simulink model "modelo_planta"  (R2023b)
settings: Solver=VariableStepAuto  StartTime=0.0  StopTime=inf  MaxStep=1e-3  RelTol=1e-3
undefined symbols (not defined in the file): ah_max, at_max, bcx, bcy, bhb, bhd, bhEb, bhm, bhwu, bt, btb, btd, btm, btw, DiscIntNeverNeededParam, g, h_vec_inicial, Hc, ih, it, J_hd_hEb, J_hm_hb, Jtd, Jtm_tb, Kcy, khwu, Ki_h, Ki_t, Kp_h, Kp_t, Kpos_h, Kpos_t, Ktw, lambda, Lh0, lh_0, magnitude, Mc_max, Mc_min, Ms, Mt, P_nom, rhd, rtd, tau_hm, tau_tm, Thb_Max, ThEb_Max, Thm_0, Thm_Max, titahm_0, titatm_0, Ts0, Ts1, Ts2, Ttb_Max, Ttm_0, Ttm_Max, vh_max_unloaded, vh_nom ... (+20)
libraries: simulink x14, vrlib x1, simulink_extras x1, dspnetwork x1
(part 1 of 2)
settings Model: PacingRate=0.500000  Creator=Nahuel  LastModifiedBy=rodri
settings SolverCC: ZeroCrossControl=DisableAll
settings DebuggingCC: UnderSpecifiedDimensionMsg=warning

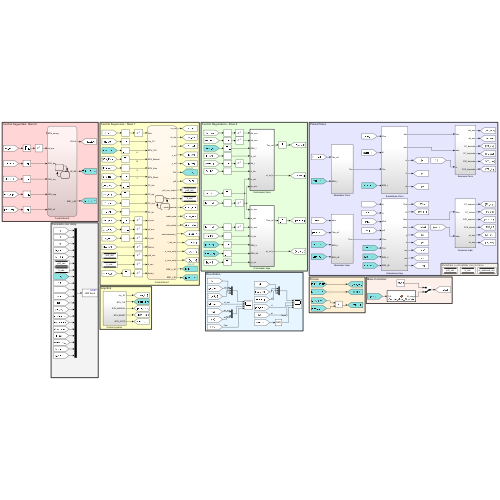
[thumbnail: Simulink's stored preview of the top-level diagram]
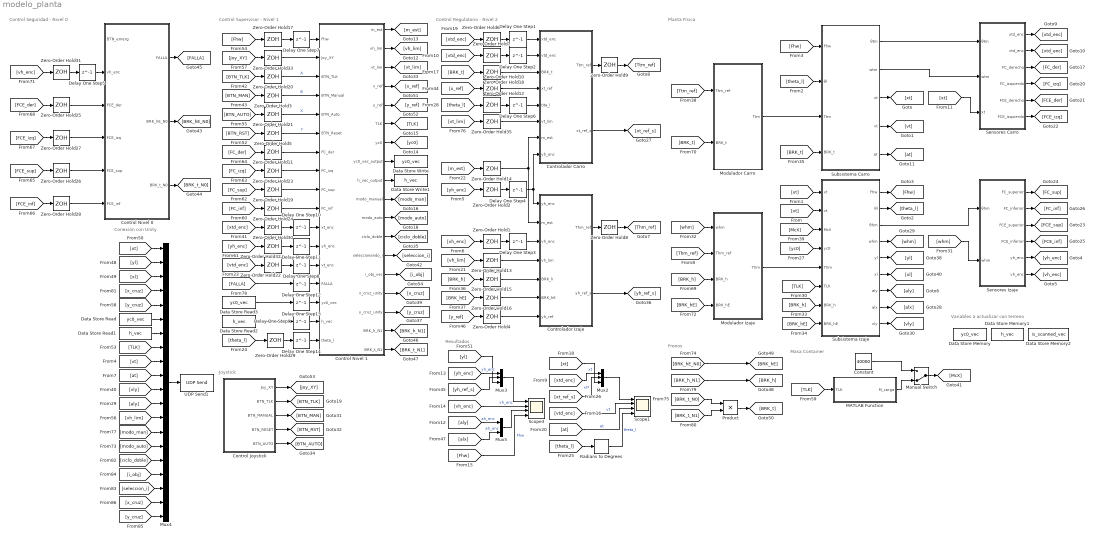
== system modelo_planta ==
  note: Joystick
  note: Frenos
  note: Control Seguridad - Nivel 0
  note: Control Regulatorio - Nivel 2
  note: Control Supervisor - Nivel 1
  note: Conexión con Unity
  note: Planta Física
  note: Resultados
  note: Variables a actualizar con terreno
  note: Masa Container
  Constant : Constant  Value=40000
  "Control Joystick " : Subsystem
  Control Nivel 0 : Stateflow chart  TreatAsAtomicUnit=on
      settings: PortSchema="{\"entries\":[{\"content\":{\"sides\":[{\"content\":{\"connectorIds\":[\"In1\",\"In4\",\"In2\",\"In5\",\"In3\",\"In6\"]},\"type\":\"ConnectorPlacement.EquallySpacedRectSide\",\"uuid\":\"72248b79-25cb-4c81-9f00-8922a9a1cf34\"},{\"content\":{\"connectorIds\":[\"Out1\",\"Out2\",\"Out3\"],\"side\":\"RIGHT\"},\"type\":\"ConnectorPlacement.EquallySpacedRectSide\",\"uuid\":\"f4bfcd12-c204-46a9-9a4b-20ccb9bfcfbb\"},{\"content\":{\"side\":\"TOP\"},\"type\":\"ConnectorPlacement.EquallySpacedRectSide\",\"uuid\":\"f84291a0-0f0e-4f0d-b220-c2febce5b448\"}]},\"type\":\"ConnectorPlacement.EquallySpacedConnector\",\"uuid\":\"3b165743-ae9e-4544-8961-e71410288a4b\"}],\"packageUris\":[\"http://schema.mathworks.com/mf0/Connector/R2020b\"],\"version\":\"1.0\"}"
  Control Nivel 1 : Stateflow chart  TreatAsAtomicUnit=on
      settings: PortSchema="{\"entries\":[{\"content\":{\"sides\":[{\"content\":{\"connectorIds\":[\"In2\",\"In4\",\"In3\",\"In5\",\"In6\",\"In7\",\"In8\",\"In10\",\"In9\",\"In11\",\"In12\",\"In13\",\"In1\",\"In14\",\"In15\",\"In16\",\"In17\"]},\"type\":\"ConnectorPlacement.EquallySpacedRectSide\",\"uuid\":\"72765c9f-68bf-44f3-92f3-3edecb9ca866\"},{\"content\":{\"connectorIds\":[\"Out1\",\"Out2\",\"Out7\",\"Out3\",\"Out4\",\"Out8\",\"Out9\",\"Out10\",\"Out11\",\"Out12\",\"Out13\",\"Out14\",\"Out15\",\"Out16\",\"Out17\",\"Out18\",\"Out5\",\"Out6\"],\"side\":\"RIGHT\"},\"type\":\"ConnectorPlacement.EquallySpacedRectSide\",\"uuid\":\"a6939ff5-eef8-44e2-80ea-5356e254e9e8\"},{\"content\":{\"side\":\"TOP\"},\"type\":\"ConnectorPlacement.EquallySpacedRectSide\",\"uuid\":\"0bd5f797-ecd4-419a-b4ec-9e10260d270a\"},{\"content\":{\"side\":\"BOTTOM\"},\"type\":\"ConnectorPlacement.EquallySpacedRectSide\",\"uuid\":\"7945275f-dab8-4c32-b5c3-f64b82fddda0\"}]},\"type\":\"ConnectorPlacement.EquallySpacedConnector\",\"uuid\":\"3d3cbadb-c70b-461a-afd4-e8d4b160ddcd\"}],\"packageUris\":[\"http://schema.mathworks.com/mf0/Connector/R2020b\"],\"version\":\"1.0\"}"
  Controlador Carro : Subsystem  TreatAsAtomicUnit=on  SystemSampleTime=Ts2
  Controlador Izaje : Subsystem  TreatAsAtomicUnit=on  SystemSampleTime=Ts2
  Data Store Memory : DataStoreMemory  DataStoreName=yc0_vec  WriteAfterWriteMsg=warning  InitialValue=yc0_vec_inicial  ShowAdditionalParam=off  OutDataTypeStr=double
  Data Store Memory1 : DataStoreMemory  DataStoreName=h_vec  WriteAfterWriteMsg=warning  InitialValue=h_vec_inicial  ShowAdditionalParam=off  OutDataTypeStr=double  Dimensions=[1,33]
  Data Store Memory2 : DataStoreMemory  DataStoreName=is_scanned_vec  WriteAfterWriteMsg=warning  InitialValue=is_scanned_vec  ShowAdditionalParam=off
  Data Store Read : DataStoreRead  DataStoreName=yc0_vec  IndexOptions=Index vector (dialog)  Indices=1  OutputSizes=1
  Data Store Read1 : DataStoreRead  DataStoreName=h_vec  IndexOptions=Index vector (dialog)  Indices=1  OutputSizes=1
  Data Store Read2 : DataStoreRead  DataStoreName=h_vec  IndexOptions=Index vector (dialog)  Indices=1  OutputSizes=1
  Data Store Read3 : DataStoreRead  DataStoreName=yc0_vec  IndexOptions=Index vector (dialog)  Indices=1  OutputSizes=1
  Data Store Write : DataStoreWrite  DataStoreName=yc0_vec  IndexOptions=Index vector (dialog)  Indices=1  OutputSizes=1
  Data Store Write1 : DataStoreWrite  DataStoreName=h_vec  IndexOptions=Index vector (dialog)  Indices=1  OutputSizes=1
  Delay One Step1 : Delay  DelayLength=1  InitialCondition=xt_0
  Delay One Step10 : Delay  DelayLength=1  InitialCondition=xt_0
  Delay One Step11 : Delay  DelayLength=1  InitialCondition=yh_0
  Delay One Step12 : Delay  DelayLength=1
  Delay One Step13 : Delay  DelayLength=1  InitialCondition=yc0_vec_inicial
  Delay One Step14 : Delay  DelayLength=1  InitialCondition=0
  Delay One Step2 : Delay  DelayLength=1  InitialCondition=vt_0
  Delay One Step3 : Delay  DelayLength=1  InitialCondition=whm_0
  Delay One Step4 : Delay  DelayLength=1  InitialCondition=yh_0
  Delay One Step5 : Delay  DelayLength=1  InitialCondition=yh_0
  Delay One Step6 : Delay  DelayLength=1  InitialCondition=0
  Delay One Step7 : Delay  DelayLength=1
  Delay One Step8 : Delay  DelayLength=1  InitialCondition=0
  Delay One Step9 : Delay  DelayLength=1  InitialCondition=h_vec_inicial
  MATLAB Function : MATLAB Function  TreatAsAtomicUnit=on
  Manual Switch : ManualSwitch  CurrentSetting=0
  Modulador Carro : Subsystem
  Modulador Izaje : Subsystem
  Mux2 : Mux  Inputs=3
  Mux3 : Mux  Inputs=3
  Mux4 : Mux  Inputs=20
  Mux5 : Mux  Inputs=2
  Product : Product
  Radians to Degrees : simulink_extras/Transformations/Radians to Degrees
  Scope1 : Scope  NumInputPorts=4
  Scope3 : Scope  NumInputPorts=4
  Sensores Carro : Subsystem
  Sensores Izaje : Subsystem
  Subsistema Carro : Subsystem
  Subsistema Izaje : Subsystem
  UDP Send1 : dspnetwork/UDP Send  remoteURL='127.0.0.1'  remotePort=1234  localURL='0.0.0.0'  localPortSource=Automatically determine  localPort=-1  sendBufferSize=8192  sampletime=-1  blockPlatform=HOST  separateLengthPort=0
  Zero-Order Hold{1..2,4,6..10,12..16,18,35} (15 alike) : ZeroOrderHold  SampleTime=Ts2
  Zero-Order Hold{3,5,11,17,19..24,29..30,32..33} (14 alike) : ZeroOrderHold  SampleTime=Ts1
  Zero-Order Hold{25..28,31} (5 alike) : ZeroOrderHold  SampleTime=Ts0
  wires:
  [Thm_ref] -> Modulador Izaje/2(Thm_ref)
  [vh_enc] -> Scope3/2  "vh_enc"
  Sensores Izaje/2(FC_inferior) -> [FC_inf]
  [x_ref] -> Zero-Order Hold10/1
  Zero-Order Hold4/1 -> Controlador Izaje/7(yh_ref)
  Delay One Step4/1 -> Controlador Izaje/1(yh_enc), Controlador Carro/8(yh_enc)
  Sensores Izaje/5(yh_enc) -> [yh_enc]
  [BRK_hE] -> Subsistema Izaje/8(BRK_hE)
  Subsistema Izaje/1(Fhw) -> [Fhw]
  [vh_enc] -> Zero-Order Hold1/1
  Controlador Izaje/1(Thm_ref) -> Zero-Order Hold8/1
  Sensores Carro/1(xtd_enc) -> [xtd_enc]
  [xt] -> Sensores Carro/3(xt)
  [BRK_h] -> Subsistema Izaje/7(BRK_h)
  Sensores Carro/4(FC_izquierdo) -> [FC_izq]
  Subsistema Izaje/4(whm) -> [whm]
  [m_est] -> Zero-Order Hold14/1
  Controlador Carro/2(xt_ref_s) -> [xt_ref_s]
  Zero-Order Hold1/1 -> Delay One Step3/1
  Zero-Order Hold2/1 -> Delay One Step4/1
  Zero-Order Hold6/1 -> Delay One Step1/1
  Subsistema Carro/2(wtm) -> Sensores Carro/2(wtm)
  Subsistema Carro/5(at) -> [at]
  [theta_l] -> Subsistema Carro/2(θl)
  [vt] -> Subsistema Izaje/2(vt)
  [xt] -> Subsistema Izaje/1(xt)
  Delay One Step1/1 -> Controlador Carro/1(xtd_enc)
  [aly] -> Mux5/1  "ah_enc"
  [vtd_enc] -> Zero-Order Hold7/1
  Sensores Carro/2(vtd_enc) -> [vtd_enc]
  Zero-Order Hold8/1 -> [Thm_ref]
  Delay One Step3/1 -> Controlador Izaje/3(vh_enc)
  [vh_lim] -> Zero-Order Hold13/1
  Delay One Step2/1 -> Controlador Carro/2(vtd_enc)
  Zero-Order Hold10/1 -> Controlador Carro/4(xt_ref)
  Subsistema Carro/3(xt) -> [xt]
  [Fhw] -> Subsistema Carro/1(Fhw)
  Sensores Carro/6(FCE_izquierdo) -> [FCE_izq]
  [yh_enc] -> Zero-Order Hold2/1
  Sensores Izaje/6(vh_enc) -> [vh_enc]
  [xtd_enc] -> Zero-Order Hold6/1
  Zero-Order Hold9/1 -> [Ttm_ref]
  Controlador Carro/1(Ttm_ref) -> Zero-Order Hold9/1
  [TLK] -> Subsistema Izaje/6(TLK)
  Subsistema Izaje/3(θhm) -> Sensores Izaje/1(θhm)
  Subsistema Carro/1(θtm) -> Sensores Carro/1(θtm)
  Sensores Izaje/4(FCE_inferior) -> [FCE_inf]
  Sensores Izaje/3(FCE_superior) -> [FCE_sup]
  Sensores Izaje/1(FC_superior) -> [FC_sup]
  Sensores Carro/5(FCE_derecho) -> [FCE_der]
  Zero-Order Hold7/1 -> Delay One Step2/1
  Subsistema Izaje/2(θl) -> [theta_l]
  [McX] -> Subsistema Izaje/3(McX)
  Subsistema Carro/4(vt) -> [vt]
  Sensores Carro/3(FC_derecho) -> [FC_der]
  [whm] -> Sensores Izaje/2(whm)
  [BRK_t] -> Subsistema Carro/4(BRK_t)
  [BRK_h] -> Zero-Order Hold15/1
  [BRK_hE] -> Zero-Order Hold16/1
  [Ttm_ref] -> Modulador Carro/1(Ttm_ref)
  [BRK_t] -> Zero-Order Hold18/1
  [yh_enc] -> Mux3/1  "yh_enc"
  [whm] -> Modulador Izaje/1(whm)
  Delay One Step6/1 -> Controlador Carro/5(tita_l)
  [theta_l] -> Zero-Order Hold12/1
  Zero-Order Hold12/1 -> Delay One Step6/1
  Modulador Izaje/1(Thm) -> Subsistema Izaje/5(Thm)
  Modulador Carro/1(Ttm) -> Subsistema Carro/3(Ttm)
  [y_ref] -> Zero-Order Hold4/1
  Mux3/1 -> Scope3/1
  Controlador Izaje/2(yh_ref_s) -> [yh_ref_s]
  [yh_ref_s] -> Mux3/2
  Subsistema Izaje/5(yl) -> [yl]
  Subsistema Izaje/6(xl) -> [xl]
  [Fhw] -> Scope3/4  "Fhw"
  Subsistema Izaje/7(aly) -> [aly]
  Subsistema Izaje/8(alx) -> [alx]
  Mux5/1 -> Scope3/3
  [alx] -> Mux5/2  "ah_enc"
  Constant/1 -> Manual Switch/1
  [yl] -> Mux3/3
  [yc0] -> Subsistema Izaje/4(yc0)
  Control Nivel 1/1(m_est) -> [m_est]
  Control Nivel 1/2(vh_lim) -> [vh_lim]
  Zero-Order Hold13/1 -> Controlador Izaje/4(vh_lim)
  Zero-Order Hold14/1 -> Controlador Izaje/2(m_est), Controlador Carro/7(m_est)
  Zero-Order Hold15/1 -> Controlador Izaje/5(BRK_h)
  Zero-Order Hold16/1 -> Controlador Izaje/6(BRK_hE)
  Zero-Order Hold17/1 -> Delay One Step7/1
  Delay One Step7/1 -> Control Nivel 1/2(Fhw)
  [Fhw] -> Zero-Order Hold17/1
  Zero-Order Hold18/1 -> Controlador Carro/3(BRK_t)
  [BTN_TLK] -> Zero-Order Hold20/1
  Zero-Order Hold20/1 -> Control Nivel 1/3(BTN_TLK)  "A"
  [at] -> Scope1/3  "at"
  [xt_ref_s] -> Mux2/2  "xt*"
  [theta_l] -> Radians to Degrees/1
  [vtd_enc] -> Scope1/2  "vt"
  [xt] -> Mux2/3
  [xtd_enc] -> Mux2/1  "xt"
  Mux2/1 -> Scope1/1
  Radians to Degrees/1 -> Scope1/4  "theta_l"
  Zero-Order Hold11/1 -> Control Nivel 1/8(FC_der)
  Zero-Order Hold19/1 -> Control Nivel 1/9(FC_sup)
  Zero-Order Hold23/1 -> Control Nivel 1/10(FC_izq)
  Zero-Order Hold24/1 -> Control Nivel 1/11(FC_inf)
  [FC_izq] -> Zero-Order Hold23/1
  [FC_der] -> Zero-Order Hold11/1
  [FC_sup] -> Zero-Order Hold19/1
  [FC_inf] -> Zero-Order Hold24/1
  Zero-Order Hold25/1 -> Control Nivel 0/2(FCE_der)
  Zero-Order Hold26/1 -> Control Nivel 0/3(FCE_sup)
  Zero-Order Hold27/1 -> Control Nivel 0/5(FCE_izq)
  Zero-Order Hold28/1 -> Control Nivel 0/6(FCE_inf)
  [FCE_der] -> Zero-Order Hold25/1
  [FCE_izq] -> Zero-Order Hold27/1
  [FCE_sup] -> Zero-Order Hold26/1
  [FCE_inf] -> Zero-Order Hold28/1
  [BRK_h] -> Modulador Izaje/3(BRK_h)
  [vh_enc] -> Zero-Order Hold31/1
  Zero-Order Hold31/1 -> Delay One Step5/1
  Delay One Step5/1 -> Control Nivel 0/4(vh_enc)
  [BRK_hE] -> Modulador Izaje/4(BRK_hE)
  [BRK_t] -> Modulador Carro/2(BRK_t)
  Control Nivel 0/2(BRK_hE_N0) -> [BRK_hE_N0]
  Control Nivel 0/3(BRK_t_N0) -> [BRK_t_N0]
  [xtd_enc] -> Zero-Order Hold30/1
  [yh_enc] -> Zero-Order Hold32/1
  Zero-Order Hold30/1 -> Delay One Step10/1
  Delay One Step10/1 -> Control Nivel 1/12(xt_enc)
  Zero-Order Hold32/1 -> Delay One Step11/1
  Delay One Step11/1 -> Control Nivel 1/13(yh_enc)
  Control Nivel 0/1(FALLA) -> [FALLA]
  [FALLA] -> Delay One Step12/1
  Control Nivel 1/5(BRK_h_N1) -> [BRK_h_N1]
  Control Nivel 1/6(BRK_t_N1) -> [BRK_t_N1]
  [BRK_t_N0] -> Product/1
  [BRK_t_N1] -> Product/2
  [BRK_h_N1] -> [BRK_h]
  [BRK_hE_N0] -> [BRK_hE]
  Product/1 -> [BRK_t]
  Control Nivel 1/3(x_ref) -> [x_ref]
  Control Nivel 1/4(y_ref) -> [y_ref]
  [BTN_MAN] -> Zero-Order Hold3/1
  Delay One Step12/1 -> Control Nivel 1/14(FALLA)
  "Control Joystick "/2(BTN_TLK) -> [BTN_TLK]
  "Control Joystick "/1(Joy_XY) -> [Joy_XY]
  [Joy_XY] -> Zero-Order Hold33/1
  Zero-Order Hold33/1 -> Control Nivel 1/4(Joy_XY)
  Zero-Order Hold35/1 -> Controlador Carro/6(vt_lim)
  Control Nivel 1/7(vt_lim) -> [vt_lim]
  [vt_lim] -> Zero-Order Hold35/1
  Control Nivel 1/8(TLK) -> [TLK]
  Control Nivel 1/9(yc0) -> [yc0]
  Data Store Read2/1 -> Delay One Step9/1
  Delay One Step9/1 -> Control Nivel 1/16(h_vec)
  Data Store Read3/1 -> Delay One Step13/1
  Delay One Step13/1 -> Control Nivel 1/15(yc0_vec)
  Control Nivel 1/10(yc0_vec_output) -> Data Store Write/1
  Control Nivel 1/11(h_vec_output) -> Data Store Write1/1
  Subsistema Izaje/9(vly) -> [vly]
  "Control Joystick "/5(BTN_AUTO) -> [BTN_AUTO]
  "Control Joystick "/4(BTN_RESET) -> [BTN_RST]
  "Control Joystick "/3(BTN_MANUAL) -> [BTN_MAN]
  Zero-Order Hold3/1 -> Control Nivel 1/5(BTN_Manual)  "B"
  [BTN_AUTO] -> Zero-Order Hold21/1
  Zero-Order Hold21/1 -> Control Nivel 1/6(BTN_Auto)  "X"
  [BTN_RST] -> Zero-Order Hold5/1
  Zero-Order Hold5/1 -> Control Nivel 1/7(BTN_Reset)  "Y"
  MATLAB Function/1(M_carga) -> Manual Switch/2
  [TLK] -> MATLAB Function/1(TLK)
  Manual Switch/1 -> [McX]
  [vh_lim] -> Mux4/13
  [at] -> Mux4/10
  [vt] -> Mux4/9
  [xt] -> Mux4/1
  Data Store Read/1 -> Mux4/6
  [vly] -> Mux4/11
  [aly] -> Mux4/12
  Data Store Read1/1 -> Mux4/7
  [yl] -> Mux4/2
  [y_cruz] -> Mux4/5
  [TLK] -> Mux4/8
  [xl] -> Mux4/3
  [x_cruz] -> Mux4/4
  Mux4/1 -> UDP Send1/1
  [vtd_enc] -> Zero-Order Hold22/1
  Zero-Order Hold22/1 -> Delay One Step8/1
  Delay One Step8/1 -> Control Nivel 1/1(vt_enc)
  [theta_l] -> Zero-Order Hold29/1
  Zero-Order Hold29/1 -> Delay One Step14/1
  Delay One Step14/1 -> Control Nivel 1/17(theta_l)
  Control Nivel 1/12(modo_manual) -> [modo_man]
  Control Nivel 1/13(modo_auto) -> [modo_auto]
  [modo_man] -> Mux4/14
  [modo_auto] -> Mux4/15
  Control Nivel 1/14(ciclo_doble) -> [ciclo_doble]
  [ciclo_doble] -> Mux4/16
  Control Nivel 1/18(y_cruz_unity) -> [y_cruz]
  Control Nivel 1/17(x_cruz_unity) -> [x_cruz]
  Control Nivel 1/15(seleccionando_i) -> [seleccion_i]
  Control Nivel 1/16(i_obj_vec) -> [i_obj]
  [i_obj] -> Mux4/17
  [seleccion_i] -> Mux4/18
  [x_cruz] -> Mux4/19
  [y_cruz] -> Mux4/20

== system modelo_planta/Control Joystick  ==
  Cast To Double : DataTypeConversion  OutDataTypeStr=double  SaturateOnIntegerOverflow=off  RndMeth=Floor
  Demux : Demux  Outputs=10
  Demux1 : Demux  Outputs=2
  Gain : Gain  Gain=-1
  Joystick Input : vrlib/Joystick Input  joyid=1  adjustports=on  forcefeed=off
  Mux : Mux  Inputs=2
  Selector : Selector  InputPortWidth=5  IndexOptions=Index vector (dialog)  Indices=[1 5]  OutputSizes=1
  Joy_XY : Outport
  BTN_TLK : Outport  Port=2
  BTN_MANUAL : Outport  Port=3
  BTN_RESET : Outport  Port=4
  BTN_AUTO : Outport  Port=5
  wires:
  Demux/1 -> BTN_TLK/1  "A"
  Joystick Input/2 -> Cast To Double/1
  Demux1/2 -> Gain/1
  Demux1/1 -> Mux/1  "LeftStick_X"
  Selector/1 -> Demux1/1
  Joystick Input/1 -> Selector/1
  Gain/1 -> Mux/2  "RightStick_Y"
  Cast To Double/1 -> Demux/1
  Demux/2 -> BTN_MANUAL/1  "B"
  Demux/3 -> BTN_AUTO/1  "X"
  Demux/4 -> BTN_RESET/1  "Y"
  Mux/1 -> Joy_XY/1

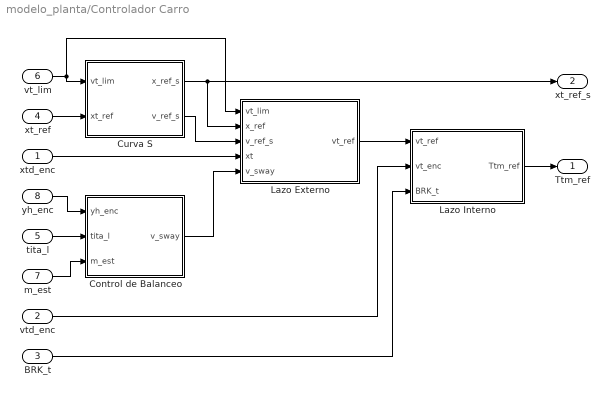
== system modelo_planta/Controlador Carro ==
  xtd_enc : Inport
  vtd_enc : Inport  Port=2
  BRK_t : Inport  Port=3
  xt_ref : Inport  Port=4
  tita_l : Inport  Port=5
  vt_lim : Inport  Port=6
  m_est : Inport  Port=7
  yh_enc : Inport  Port=8
  Control de Balanceo : Subsystem
  Curva S : Subsystem
  Lazo Externo : Subsystem
  Lazo Interno : Subsystem
  Ttm_ref : Outport
  xt_ref_s : Outport  Port=2
  wires:
  Lazo Externo/1(vt_ref) -> Lazo Interno/1(vt_ref)
  vtd_enc/1 -> Lazo Interno/2(vt_enc)
  xt_ref/1 -> Curva S/2(xt_ref)
  Curva S/1(x_ref_s) -> Lazo Externo/2(x_ref), xt_ref_s/1
  xtd_enc/1 -> Lazo Externo/4(xt)
  Control de Balanceo/1(v_sway) -> Lazo Externo/5(v_sway)
  BRK_t/1 -> Lazo Interno/3(BRK_t)
  Lazo Interno/1(Ttm_ref) -> Ttm_ref/1
  yh_enc/1 -> Control de Balanceo/1(yh_enc)
  tita_l/1 -> Control de Balanceo/2(tita_l)
  vt_lim/1 -> Curva S/1(vt_lim), Lazo Externo/1(vt_lim)
  Curva S/2(v_ref_s) -> Lazo Externo/3(v_ref_s)
  m_est/1 -> Control de Balanceo/3(m_est)

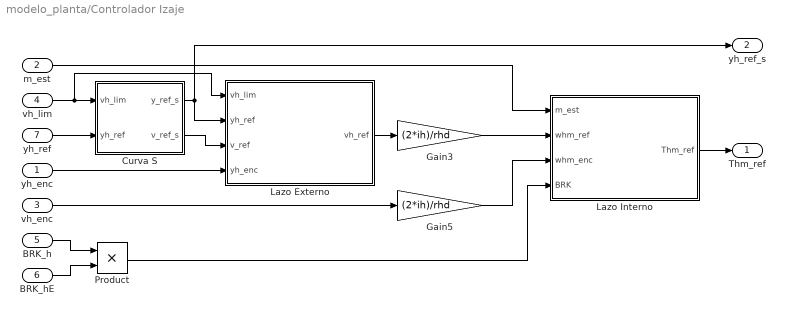
== system modelo_planta/Controlador Izaje ==
  yh_enc : Inport
  m_est : Inport  Port=2
  vh_enc : Inport  Port=3
  vh_lim : Inport  Port=4
  BRK_h : Inport  Port=5
  BRK_hE : Inport  Port=6
  yh_ref : Inport  Port=7
  Curva S : Subsystem
  Gain3 : Gain  Gain=(2*ih)/rhd
  Gain5 : Gain  Gain=(2*ih)/rhd
  Lazo Externo : Subsystem  TreatAsAtomicUnit=on  SystemSampleTime=Ts2
  Lazo Interno : Subsystem  TreatAsAtomicUnit=on  SystemSampleTime=Ts2
  Product : Product
  Thm_ref : Outport
  yh_ref_s : Outport  Port=2
  wires:
  Lazo Externo/1(vh_ref) -> Gain3/1
  m_est/1 -> Lazo Interno/1(m_est)
  vh_enc/1 -> Gain5/1
  yh_enc/1 -> Lazo Externo/4(yh_enc)
  Gain5/1 -> Lazo Interno/3(whm_enc)
  yh_ref/1 -> Curva S/2(yh_ref)
  Gain3/1 -> Lazo Interno/2(whm_ref)
  BRK_h/1 -> Product/1
  BRK_hE/1 -> Product/2
  vh_lim/1 -> Lazo Externo/1(vh_lim), Curva S/1(vh_lim)
  Product/1 -> Lazo Interno/4(BRK)
  Lazo Interno/1(Thm_ref) -> Thm_ref/1
  Curva S/1(y_ref_s) -> Lazo Externo/2(yh_ref), yh_ref_s/1
  Curva S/2(v_ref_s) -> Lazo Externo/3(v_ref)

== system modelo_planta/Modulador Carro ==
  Ttm_ref : Inport
  BRK_t : Inport  Port=2
  Constant : Constant  Value=Ttm_Max
  Gain1 : Gain  Gain=-1
  Gain2 : Gain  Gain=1/tau_tm
  Integrator : Integrator  InitialCondition=Ttm_0
  Product : Product
  Saturation Dynamic : simulink/Discontinuities/Saturation Dynamic  OutMin=[]  OutMax=[]  OutDataTypeStr=Inherit: Same as second input  OutDataType=fixdt(1, 16)  OutScaling=2^-10  DoSatur=off
  Sum : Sum  Inputs=|+-
  Ttm : Outport
  wires:
  Constant/1 -> Saturation Dynamic/1, Gain1/1
  Gain1/1 -> Saturation Dynamic/3
  Saturation Dynamic/1 -> Sum/1  "Ttm_lim"
  Sum/1 -> Gain2/1
  Gain2/1 -> Integrator/1
  Integrator/1 -> Ttm/1, Sum/2
  Ttm_ref/1 -> Product/1
  BRK_t/1 -> Product/2
  Product/1 -> Saturation Dynamic/2

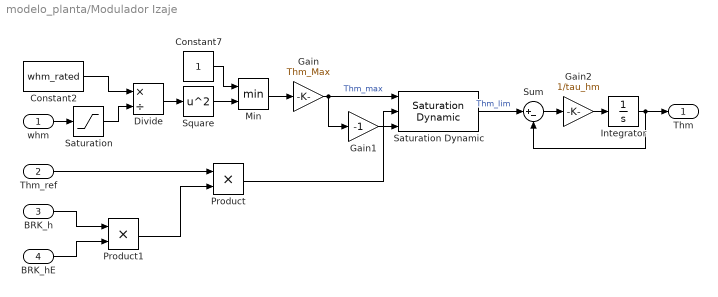
== system modelo_planta/Modulador Izaje ==
  whm : Inport
  Thm_ref : Inport  Port=2
  BRK_h : Inport  Port=3
  BRK_hE : Inport  Port=4
  Constant2 : Constant  Value=whm_rated
  Constant7 : Constant
  Divide : Product  Inputs=*/
  Gain : Gain  Gain=Thm_Max
  Gain1 : Gain  Gain=-1
  Gain2 : Gain  Gain=1/tau_hm
  Integrator : Integrator  InitialCondition=Thm_0
  Min : MinMax  Inputs=2
  Product : Product
  Product1 : Product
  Saturation : Saturate  UpperLimit=inf  LowerLimit=whm_rated
  Saturation Dynamic : simulink/Discontinuities/Saturation Dynamic  OutMin=[]  OutMax=[]  OutDataTypeStr=Inherit: Same as second input  OutDataType=fixdt(1, 16)  OutScaling=2^-10  DoSatur=off
  Square : Math  Operator=square
  Sum : Sum  Inputs=|+-
  Thm : Outport
  wires:
  Constant2/1 -> Divide/1
  Min/1 -> Gain/1
  Constant7/1 -> Min/1
  Gain/1 -> Gain1/1, Saturation Dynamic/1  "Thm_max"
  Saturation/1 -> Divide/2
  Square/1 -> Min/2
  Divide/1 -> Square/1
  whm/1 -> Saturation/1
  Gain1/1 -> Saturation Dynamic/3
  Saturation Dynamic/1 -> Sum/1  "Thm_lim"
  Sum/1 -> Gain2/1
  Gain2/1 -> Integrator/1
  Integrator/1 -> Thm/1, Sum/2
  Thm_ref/1 -> Product/1
  BRK_h/1 -> Product1/1
  Product/1 -> Saturation Dynamic/2
  BRK_hE/1 -> Product1/2
  Product1/1 -> Product/2

== system modelo_planta/Sensores Carro ==
  θtm : Inport
  wtm : Inport  Port=2
  xt : Inport  Port=3
  Encoder Carro : Subsystem
  Fines de carrera carro (rieles) : Subsystem
  xtd_enc : Outport
  vtd_enc : Outport  Port=2
  FC_derecho : Outport  Port=3
  FC_izquierdo : Outport  Port=4
  FCE_derecho : Outport  Port=5
  FCE_izquierdo : Outport  Port=6
  wires:
  Encoder Carro/1(xtd_enc) -> xtd_enc/1
  Fines de carrera carro (rieles)/1(FC_derecho) -> FC_derecho/1
  θtm/1 -> Encoder Carro/1(θtm)
  Fines de carrera carro (rieles)/2(FC_izquierdo) -> FC_izquierdo/1
  Encoder Carro/2(vtd_enc) -> vtd_enc/1
  Fines de carrera carro (rieles)/3(FCE_derecho) -> FCE_derecho/1
  Fines de carrera carro (rieles)/4(FCE_izquierdo) -> FCE_izquierdo/1
  xt/1 -> Fines de carrera carro (rieles)/1(xt)
  wtm/1 -> Encoder Carro/2(wtm)

== system modelo_planta/Sensores Izaje ==
  θhm : Inport
  whm : Inport  Port=2
  Encoder Izaje : Subsystem
  Fines de carrera izaje (tambor) : Subsystem
  FC_superior : Outport
  FC_inferior : Outport  Port=2
  FCE_superior : Outport  Port=3
  FCE_inferior : Outport  Port=4
  yh_enc : Outport  Port=5
  vh_enc : Outport  Port=6
  wires:
  Fines de carrera izaje (tambor)/1(FC_superior) -> FC_superior/1
  whm/1 -> Encoder Izaje/2(whm)
  Fines de carrera izaje (tambor)/4(FCE_inferior) -> FCE_inferior/1
  Fines de carrera izaje (tambor)/2(FC_inferior) -> FC_inferior/1
  Encoder Izaje/2(yh_enc) -> Fines de carrera izaje (tambor)/1(y_enc), yh_enc/1
  θhm/1 -> Encoder Izaje/1(θhm)
  Fines de carrera izaje (tambor)/3(FCE_superior) -> FCE_superior/1
  Encoder Izaje/1(vh_enc) -> vh_enc/1

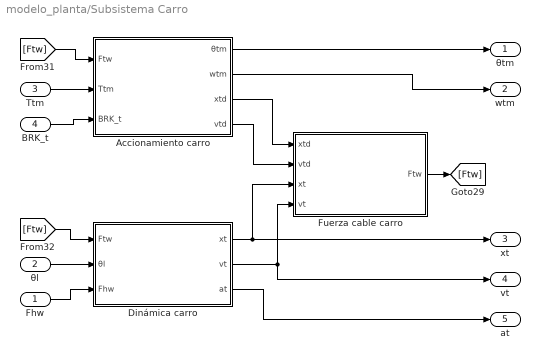
== system modelo_planta/Subsistema Carro ==
  Fhw : Inport
  θl : Inport  Port=2
  Ttm : Inport  Port=3
  BRK_t : Inport  Port=4
  Accionamiento carro : Subsystem
  Dinámica carro : Subsystem
  Fuerza cable carro : Subsystem
  θtm : Outport
  wtm : Outport  Port=2
  xt : Outport  Port=3
  vt : Outport  Port=4
  at : Outport  Port=5
  wires:
  [Ftw] -> Accionamiento carro/1(Ftw)
  Accionamiento carro/1(θtm) -> θtm/1
  Dinámica carro/1(xt) -> Fuerza cable carro/3(xt), xt/1
  BRK_t/1 -> Accionamiento carro/3(BRK_t)
  [Ftw] -> Dinámica carro/1(Ftw)
  θl/1 -> Dinámica carro/2(θl)
  Ttm/1 -> Accionamiento carro/2(Ttm)
  Fuerza cable carro/1(Ftw) -> [Ftw]
  Dinámica carro/2(vt) -> Fuerza cable carro/4(vt), vt/1
  Accionamiento carro/3(xtd) -> Fuerza cable carro/1(xtd)
  Accionamiento carro/2(wtm) -> wtm/1
  Accionamiento carro/4(vtd) -> Fuerza cable carro/2(vtd)
  Fhw/1 -> Dinámica carro/3(Fhw)
  Dinámica carro/3(at) -> at/1

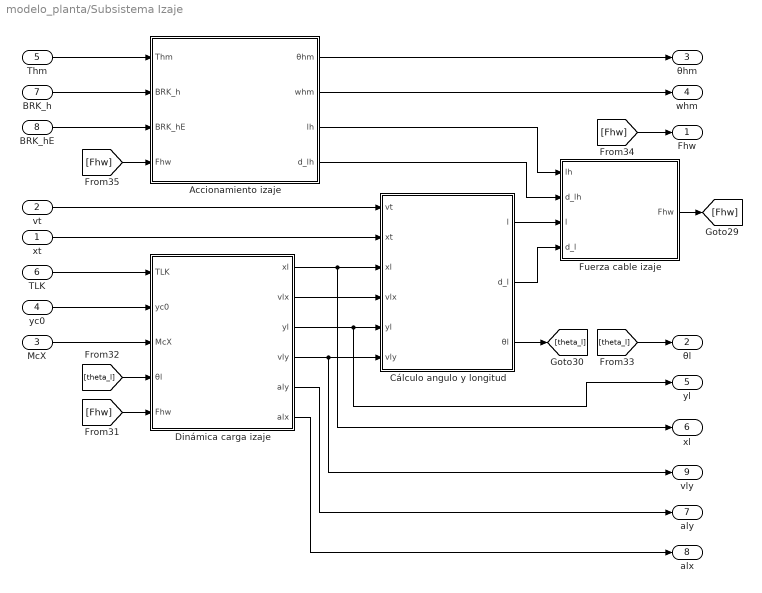
== system modelo_planta/Subsistema Izaje ==
  xt : Inport
  vt : Inport  Port=2
  McX : Inport  Port=3
  yc0 : Inport  Port=4
  Thm : Inport  Port=5
  TLK : Inport  Port=6
  BRK_h : Inport  Port=7
  BRK_hE : Inport  Port=8
  Accionamiento izaje : Subsystem
  Cálculo angulo y longitud : Subsystem
  Dinámica carga izaje : Subsystem
  Fuerza cable izaje : Subsystem
  Fhw : Outport
  θl : Outport  Port=2
  θhm : Outport  Port=3
  whm : Outport  Port=4
  yl : Outport  Port=5
  xl : Outport  Port=6
  aly : Outport  Port=7
  alx : Outport  Port=8
  vly : Outport  Port=9
  wires:
  vt/1 -> Cálculo angulo y longitud/1(vt)
  Accionamiento izaje/3(lh) -> Fuerza cable izaje/1(lh)
  yc0/1 -> Dinámica carga izaje/2(yc0)
  McX/1 -> Dinámica carga izaje/3(McX)
  Dinámica carga izaje/4(vly) -> vly/1, Cálculo angulo y longitud/6(vly)
  [Fhw] -> Accionamiento izaje/4(Fhw)
  [theta_l] -> Dinámica carga izaje/4(θl)
  Cálculo angulo y longitud/3(θl) -> [theta_l]
  xt/1 -> Cálculo angulo y longitud/2(xt)
  BRK_h/1 -> Accionamiento izaje/2(BRK_h)
  Dinámica carga izaje/1(xl) -> Cálculo angulo y longitud/3(xl), xl/1
  Dinámica carga izaje/2(vlx) -> Cálculo angulo y longitud/4(vlx)
  Fuerza cable izaje/1(Fhw) -> [Fhw]
  Cálculo angulo y longitud/1(l) -> Fuerza cable izaje/3(l)
  Accionamiento izaje/1(θhm) -> θhm/1
  [theta_l] -> θl/1
  TLK/1 -> Dinámica carga izaje/1(TLK)
  [Fhw] -> Dinámica carga izaje/5(Fhw)
  Accionamiento izaje/2(whm) -> whm/1
  BRK_hE/1 -> Accionamiento izaje/3(BRK_hE)
  Thm/1 -> Accionamiento izaje/1(Thm)
  Dinámica carga izaje/3(yl) -> yl/1, Cálculo angulo y longitud/5(yl)
  Cálculo angulo y longitud/2(d_l) -> Fuerza cable izaje/4(d_l)
  Accionamiento izaje/4(d_lh) -> Fuerza cable izaje/2(d_lh)
  Dinámica carga izaje/5(aly) -> aly/1
  Dinámica carga izaje/6(alx) -> alx/1
  [Fhw] -> Fhw/1

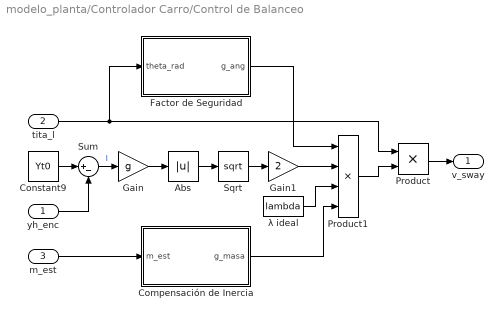
== system modelo_planta/Controlador Carro/Control de Balanceo ==
  yh_enc : Inport
  tita_l : Inport  Port=2
  m_est : Inport  Port=3
  Abs : Abs  SaturateOnIntegerOverflow=off
  Compensación de Inercia : MATLAB Function  TreatAsAtomicUnit=on
  Constant9 : Constant  Value=Yt0
  Factor de Seguridad : MATLAB Function  TreatAsAtomicUnit=on
  Gain : Gain  Gain=g
  Gain1 : Gain  Gain=2
  Product : Product
  Product1 : Product  Inputs=4
  Sqrt : Sqrt
  Sum : Sum  Inputs=|+-
  λ ideal : Constant  Value=lambda
  v_sway : Outport
  wires:
  Gain1/1 -> Product1/2
  yh_enc/1 -> Sum/2
  Product/1 -> v_sway/1
  tita_l/1 -> Factor de Seguridad/1(theta_rad), Product/1
  Sum/1 -> Gain/1  "l"
  Constant9/1 -> Sum/1
  Sqrt/1 -> Gain1/1
  Gain/1 -> Abs/1
  Abs/1 -> Sqrt/1
  m_est/1 -> Compensación de Inercia/1(m_est)
  Compensación de Inercia/1(g_masa) -> Product1/4
  Product1/1 -> Product/2
  Factor de Seguridad/1(g_ang) -> Product1/1
  λ ideal/1 -> Product1/3

== system modelo_planta/Controlador Carro/Curva S ==
  vt_lim : Inport
  xt_ref : Inport  Port=2
  Delay : Delay  DelayLength=1  InitialCondition=xt_0
  Discrete-Time Integrator1 : DiscreteIntegrator  IntegratorMethod=Integration: Trapezoidal  InitialCondition=xt_0  SampleTime=-1  ICPrevOutput=DiscIntNeverNeededParam  ICPrevScaledInput=DiscIntNeverNeededParam
  Gain1 : Gain  Gain=-1
  MATLAB Function : MATLAB Function  TreatAsAtomicUnit=on
  Rate Limiter : RateLimiter  RisingSlewLimit=at_max  FallingSlewLimit=-at_max  SampleTimeMode=inherited
  Saturation Dynamic : simulink/Discontinuities/Saturation Dynamic  OutMin=[]  OutMax=[]  OutDataTypeStr=Inherit: Same as second input  OutDataType=fixdt(1, 16)  OutScaling=2^-10  DoSatur=off
  Sum : Sum  Inputs=|+-
  x_ref_s : Outport
  v_ref_s : Outport  Port=2
  wires:
  MATLAB Function/1(vt_cmd) -> Saturation Dynamic/2  "vt_cmd"
  Discrete-Time Integrator1/1 -> x_ref_s/1, Delay/1
  Rate Limiter/1 -> v_ref_s/1, Discrete-Time Integrator1/1
  Sum/1 -> MATLAB Function/1(error_pos)
  Saturation Dynamic/1 -> Rate Limiter/1  "vt_ref"
  xt_ref/1 -> Sum/1
  Delay/1 -> Sum/2
  vt_lim/1 -> Saturation Dynamic/1, Gain1/1
  Gain1/1 -> Saturation Dynamic/3

== system modelo_planta/Controlador Carro/Lazo Externo ==
  vt_lim : Inport
  x_ref : Inport  Port=2
  v_ref_s : Inport  Port=3
  xt : Inport  Port=4
  v_sway : Inport  Port=5
  Gain : Gain  Gain=Kpos_t
  Gain1 : Gain  Gain=0.5
  Gain2 : Gain  Gain=-1
  Rate Limiter : RateLimiter  RisingSlewLimit=at_max  FallingSlewLimit=-at_max  SampleTimeMode=inherited
  Saturation Dynamic : simulink/Discontinuities/Saturation Dynamic  OutMin=[]  OutMax=[]  OutDataTypeStr=Inherit: Same as second input  OutDataType=fixdt(1, 16)  OutScaling=2^-10  DoSatur=off
  Sum1 : Sum  Inputs=+++
  Sum3 : Sum  Inputs=|+-
  vt_ref : Outport
  wires:
  xt/1 -> Sum3/2
  x_ref/1 -> Sum3/1
  Sum3/1 -> Gain/1  "e_x"
  Gain/1 -> Sum1/1
  v_ref_s/1 -> Gain1/1
  Gain1/1 -> Sum1/3
  v_sway/1 -> Sum1/2
  Saturation Dynamic/1 -> Rate Limiter/1
  Rate Limiter/1 -> vt_ref/1
  Gain2/1 -> Saturation Dynamic/3
  vt_lim/1 -> Saturation Dynamic/1, Gain2/1
  Sum1/1 -> Saturation Dynamic/2  "vt_cmd"

== system modelo_planta/Controlador Carro/Lazo Interno ==
  vt_ref : Inport
  vt_enc : Inport  Port=2
  BRK_t : Inport  Port=3
  Discrete-Time Integrator : DiscreteIntegrator  IntegratorMethod=Integration: Trapezoidal  ExternalReset=level  SampleTime=-1  ICPrevOutput=DiscIntNeverNeededParam  ICPrevScaledInput=DiscIntNeverNeededParam
  Gain5 : Gain  Gain=Ki_t
  Gain6 : Gain  Gain=Kp_t
  NOT : Logic  Operator=NOT  IconShape=distinctive  AllPortsSameDT=off  OutDataTypeStr=boolean
  Sum6 : Sum  Inputs=+-
  Sum7 : Sum  Inputs=++|
  Ttm_ref : Outport
  wires:
  Sum6/1 -> Gain6/1, Discrete-Time Integrator/1  "e_v"
  Sum7/1 -> Ttm_ref/1
  Gain5/1 -> Sum7/2
  vt_ref/1 -> Sum6/1
  Gain6/1 -> Sum7/1
  vt_enc/1 -> Sum6/2
  Discrete-Time Integrator/1 -> Gain5/1
  BRK_t/1 -> NOT/1
  NOT/1 -> Discrete-Time Integrator/2

== system modelo_planta/Controlador Izaje/Curva S ==
  vh_lim : Inport
  yh_ref : Inport  Port=2
  Delay : Delay  DelayLength=1  InitialCondition=yh_0
  Discrete-Time Integrator : DiscreteIntegrator  IntegratorMethod=Integration: Trapezoidal  InitialCondition=yh_0  SampleTime=-1  ICPrevOutput=DiscIntNeverNeededParam  ICPrevScaledInput=DiscIntNeverNeededParam
  Gain1 : Gain  Gain=-1
  MATLAB Function : MATLAB Function  TreatAsAtomicUnit=on
  Rate Limiter : RateLimiter  RisingSlewLimit=ah_max  FallingSlewLimit=-ah_max  SampleTimeMode=inherited
  Saturation Dynamic : simulink/Discontinuities/Saturation Dynamic  OutMin=[]  OutMax=[]  OutDataTypeStr=Inherit: Same as second input  OutDataType=fixdt(1, 16)  OutScaling=2^-10  DoSatur=off
  Sum : Sum  Inputs=|+-
  y_ref_s : Outport
  v_ref_s : Outport  Port=2
  wires:
  MATLAB Function/1(vh_cmd) -> Saturation Dynamic/2  "vh_cmd"
  Discrete-Time Integrator/1 -> y_ref_s/1, Delay/1
  Sum/1 -> MATLAB Function/1(error_pos)
  vh_lim/1 -> Gain1/1, Saturation Dynamic/1
  Gain1/1 -> Saturation Dynamic/3
  Saturation Dynamic/1 -> Rate Limiter/1  "vh_ref"
  yh_ref/1 -> Sum/1
  Delay/1 -> Sum/2
  Rate Limiter/1 -> v_ref_s/1, Discrete-Time Integrator/1

== system modelo_planta/Controlador Izaje/Lazo Externo ==
  vh_lim : Inport
  yh_ref : Inport  Port=2
  v_ref : Inport  Port=3
  yh_enc : Inport  Port=4
  Gain : Gain  Gain=0.5
  Gain1 : Gain  Gain=-1
  Kpos : Gain  Gain=Kpos_h
  Rate Limiter : RateLimiter  RisingSlewLimit=ah_max  FallingSlewLimit=-ah_max  SampleTimeMode=inherited
  Saturation Dynamic : simulink/Discontinuities/Saturation Dynamic  OutMin=[]  OutMax=[]  OutDataTypeStr=Inherit: Same as second input  OutDataType=fixdt(1, 16)  OutScaling=2^-10  DoSatur=off
  Sum : Sum  Inputs=|+-
  Sum1 : Sum  Inputs=|++
  vh_ref : Outport
  wires:
  yh_ref/1 -> Sum/1
  yh_enc/1 -> Sum/2
  Kpos/1 -> Sum1/1
  Sum/1 -> Kpos/1
  v_ref/1 -> Gain/1
  Gain/1 -> Sum1/2
  Sum1/1 -> Saturation Dynamic/2
  Saturation Dynamic/1 -> Rate Limiter/1
  vh_lim/1 -> Gain1/1, Saturation Dynamic/1
  Gain1/1 -> Saturation Dynamic/3
  Rate Limiter/1 -> vh_ref/1

== system modelo_planta/Controlador Izaje/Lazo Interno ==
  m_est : Inport
  whm_ref : Inport  Port=2
  whm_enc : Inport  Port=3
  BRK : Inport  Port=4
  Discrete-Time Integrator : DiscreteIntegrator  IntegratorMethod=Integration: Trapezoidal  ExternalReset=level  SampleTime=-1  ICPrevOutput=DiscIntNeverNeededParam  ICPrevScaledInput=DiscIntNeverNeededParam
  Gain : Gain  Gain=Ki_h
  Gain1 : Gain  Gain=Kp_h
  Gain2 : Gain  Gain=g*rhd/(2*ih)
  NOT : Logic  Operator=NOT  IconShape=distinctive  AllPortsSameDT=off  OutDataTypeStr=boolean
  Sum1 : Sum  Inputs=+-
  Sum4 : Sum  Inputs=|++
  Sum5 : Sum  Inputs=|++
  Thm_ref : Outport
  wires:
  Gain1/1 -> Sum4/1
  Sum1/1 -> Discrete-Time Integrator/1, Gain1/1  "e_wh"
  whm_enc/1 -> Sum1/2
  Gain2/1 -> Sum5/2  "Tg_ff"
  Sum5/1 -> Thm_ref/1  "Thm_ref"
  Sum4/1 -> Sum5/1  "T_PID"
  whm_ref/1 -> Sum1/1
  m_est/1 -> Gain2/1
  Discrete-Time Integrator/1 -> Gain/1
  Gain/1 -> Sum4/2
  NOT/1 -> Discrete-Time Integrator/2
  BRK/1 -> NOT/1

== system modelo_planta/Sensores Carro/Encoder Carro ==
  θtm : Inport
  wtm : Inport  Port=2
  Gain : Gain  Gain=rtd/it
  Gain1 : Gain  Gain=rtd/it
  xtd_enc : Outport
  vtd_enc : Outport  Port=2
  wires:
  Gain1/1 -> vtd_enc/1
  Gain/1 -> xtd_enc/1
  wtm/1 -> Gain1/1
  θtm/1 -> Gain/1

== system modelo_planta/Sensores Carro/Fines de carrera carro (rieles) ==
  xt : Inport
  Compare To Constant : simulink/Logic and Bit Operations/Compare To Constant  relop=>=  const=xt_max  OutDataTypeStr=boolean
  Compare To Constant1 : simulink/Logic and Bit Operations/Compare To Constant  relop=>=  const=xt_max+0.5  OutDataTypeStr=boolean
  Compare To Constant2 : simulink/Logic and Bit Operations/Compare To Constant  relop=<=  const=xt_min  OutDataTypeStr=boolean
  Compare To Constant3 : simulink/Logic and Bit Operations/Compare To Constant  relop=<=  const=xt_min-0.5  OutDataTypeStr=boolean
  FC_derecho : Outport
  FC_izquierdo : Outport  Port=2
  FCE_derecho : Outport  Port=3
  FCE_izquierdo : Outport  Port=4
  wires:
  Compare To Constant2/1 -> FC_izquierdo/1
  xt/1 -> Compare To Constant/1, Compare To Constant1/1, Compare To Constant2/1, Compare To Constant3/1
  Compare To Constant3/1 -> FCE_izquierdo/1
  Compare To Constant1/1 -> FCE_derecho/1
  Compare To Constant/1 -> FC_derecho/1

== system modelo_planta/Sensores Izaje/Encoder Izaje ==
  θhm : Inport
  whm : Inport  Port=2
  Gain1 : Gain  Gain=rhd/(2*ih)
  Gain3 : Gain  Gain=rhd/(2*ih)
  vh_enc : Outport
  yh_enc : Outport  Port=2
  wires:
  Gain1/1 -> vh_enc/1
  θhm/1 -> Gain3/1
  whm/1 -> Gain1/1
  Gain3/1 -> yh_enc/1

== system modelo_planta/Sensores Izaje/Fines de carrera izaje (tambor) ==
  y_enc : Inport
  Compare To Constant4 : simulink/Logic and Bit Operations/Compare To Constant  relop=>=  const=yh_max  OutDataTypeStr=boolean
  Compare To Constant5 : simulink/Logic and Bit Operations/Compare To Constant  relop=>=  const=yh_max+0.5  OutDataTypeStr=boolean
  Compare To Constant6 : simulink/Logic and Bit Operations/Compare To Constant  relop=<=  const=yh_min  OutDataTypeStr=boolean
  Compare To Constant7 : simulink/Logic and Bit Operations/Compare To Constant  relop=<=  const=yh_min-0.5  OutDataTypeStr=boolean
  FC_superior : Outport
  FC_inferior : Outport  Port=2
  FCE_superior : Outport  Port=3
  FCE_inferior : Outport  Port=4
  wires:
  Compare To Constant7/1 -> FCE_inferior/1
  y_enc/1 -> Compare To Constant7/1, Compare To Constant6/1, Compare To Constant4/1, Compare To Constant5/1
  Compare To Constant6/1 -> FC_inferior/1
  Compare To Constant5/1 -> FCE_superior/1
  Compare To Constant4/1 -> FC_superior/1

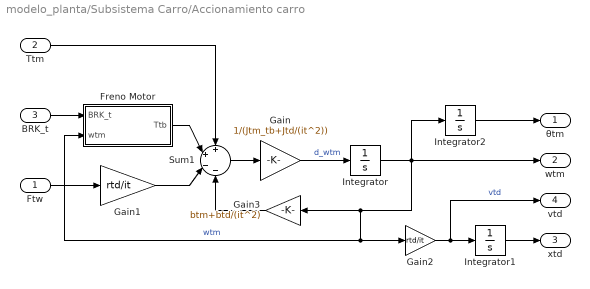
== system modelo_planta/Subsistema Carro/Accionamiento carro ==
  Ftw : Inport
  Ttm : Inport  Port=2
  BRK_t : Inport  Port=3
  Freno Motor : Subsystem
  Gain : Gain  Gain=1/(Jtm_tb+Jtd/(it^2))
  Gain1 : Gain  Gain=rtd/it
  Gain2 : Gain  Gain=rtd/it
  Gain3 : Gain  Gain=btm+btd/(it^2)
  Integrator : Integrator  InitialCondition=wtm_0
  Integrator1 : Integrator  InitialCondition=xtd_0
  Integrator2 : Integrator  InitialCondition=titatm_0
  Sum1 : Sum  Inputs=++--
  θtm : Outport
  wtm : Outport  Port=2
  xtd : Outport  Port=3
  vtd : Outport  Port=4
  wires:
  Sum1/1 -> Gain/1
  Integrator/1 -> Gain2/1, Freno Motor/2(wtm), Gain3/1, Integrator2/1, wtm/1  "wtm"
  Gain2/1 -> Integrator1/1, vtd/1  "vtd"
  Ttm/1 -> Sum1/1
  Gain/1 -> Integrator/1  "d_wtm"
  BRK_t/1 -> Freno Motor/1(BRK_t)
  Integrator1/1 -> xtd/1
  Ftw/1 -> Gain1/1
  Gain1/1 -> Sum1/3
  Freno Motor/1(Ttb) -> Sum1/2
  Gain3/1 -> Sum1/4
  Integrator2/1 -> θtm/1

== system modelo_planta/Subsistema Carro/Dinámica carro ==
  Ftw : Inport
  θl : Inport  Port=2
  Fhw : Inport  Port=3
  Gain : Gain  Gain=2
  Gain1 : Gain  Gain=1/Mt
  Gain2 : Gain  Gain=bt
  Integrator : Integrator  InitialCondition=vt_0
  Integrator1 : Integrator  InitialCondition=xt_0
  Product : Product
  Sin : Trigonometry
  Sum : Sum  Inputs=++-
  xt : Outport
  vt : Outport  Port=2
  at : Outport  Port=3
  wires:
  Gain1/1 -> at/1, Integrator/1  "dot_vt"
  Integrator/1 -> Gain2/1, vt/1, Integrator1/1  "vt"
  Gain2/1 -> Sum/3
  Sum/1 -> Gain1/1
  Integrator1/1 -> xt/1  "xt"
  Fhw/1 -> Gain/1
  Gain/1 -> Product/2
  θl/1 -> Sin/1
  Sin/1 -> Product/1
  Product/1 -> Sum/2  "F_coupling"
  Ftw/1 -> Sum/1

== system modelo_planta/Subsistema Carro/Fuerza cable carro ==
  xtd : Inport
  vtd : Inport  Port=2
  xt : Inport  Port=3
  vt : Inport  Port=4
  Gain : Gain  Gain=Ktw
  Gain1 : Gain  Gain=btw
  Sum : Sum  Inputs=+-
  Sum1 : Sum
  Sum2 : Sum  Inputs=+-
  Ftw : Outport
  wires:
  xtd/1 -> Sum/1
  Gain1/1 -> Sum1/2
  Sum/1 -> Gain/1
  xt/1 -> Sum/2
  Sum2/1 -> Gain1/1
  Gain/1 -> Sum1/1
  vt/1 -> Sum2/2
  Sum1/1 -> Ftw/1  "Ftw"
  vtd/1 -> Sum2/1

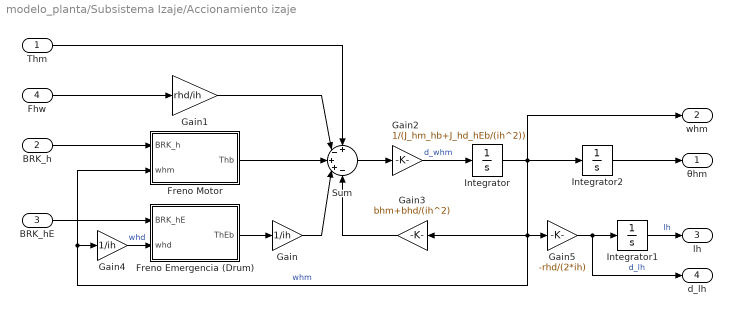
== system modelo_planta/Subsistema Izaje/Accionamiento izaje ==
  Thm : Inport
  BRK_h : Inport  Port=2
  BRK_hE : Inport  Port=3
  Fhw : Inport  Port=4
  Freno Emergencia (Drum) : Subsystem
  Freno Motor : Subsystem
  Gain : Gain  Gain=1/ih
  Gain1 : Gain  Gain=rhd/ih
  Gain2 : Gain  Gain=1/(J_hm_hb+J_hd_hEb/(ih^2))
  Gain3 : Gain  Gain=bhm+bhd/(ih^2)
  Gain4 : Gain  Gain=1/ih
  Gain5 : Gain  Gain=-rhd/(2*ih)
  Integrator : Integrator  InitialCondition=whm_0
  Integrator1 : Integrator  InitialCondition=lh_0
  Integrator2 : Integrator  InitialCondition=titahm_0
  Sum : Sum  Inputs=+-++-
  θhm : Outport
  whm : Outport  Port=2
  lh : Outport  Port=3
  d_lh : Outport  Port=4
  wires:
  Gain5/1 -> d_lh/1, Integrator1/1  "d_lh"
  Integrator/1 -> Gain3/1, Freno Motor/2(whm), Gain4/1, Gain5/1, whm/1, Integrator2/1  "whm"
  Freno Emergencia (Drum)/1(ThEb) -> Gain/1
  Gain3/1 -> Sum/5
  BRK_h/1 -> Freno Motor/1(BRK_h)
  Gain/1 -> Sum/4
  Gain2/1 -> Integrator/1  "d_whm"
  Sum/1 -> Gain2/1
  Gain4/1 -> Freno Emergencia (Drum)/2(whd)  "whd"
  BRK_hE/1 -> Freno Emergencia (Drum)/1(BRK_hE)
  Fhw/1 -> Gain1/1
  Freno Motor/1(Thb) -> Sum/3
  Gain1/1 -> Sum/2
  Integrator1/1 -> lh/1  "lh"
  Integrator2/1 -> θhm/1
  Thm/1 -> Sum/1

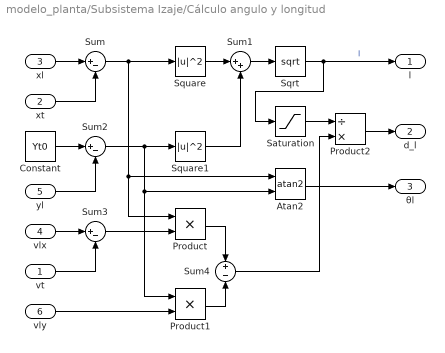
== system modelo_planta/Subsistema Izaje/Cálculo angulo y longitud ==
  vt : Inport
  xt : Inport  Port=2
  xl : Inport  Port=3
  vlx : Inport  Port=4
  yl : Inport  Port=5
  vly : Inport  Port=6
  Atan2 : Trigonometry  Operator=atan2
  Constant : Constant  Value=Yt0
  Product : Product
  Product1 : Product
  Product2 : Product  Inputs=/*
  Saturation : Saturate  UpperLimit=inf  LowerLimit=0.1
  Sqrt : Sqrt
  Square : Math  Operator=magnitude^2
  Square1 : Math  Operator=magnitude^2
  Sum : Sum  Inputs=|+-
  Sum1 : Sum  Inputs=|++
  Sum2 : Sum  Inputs=|+-
  Sum3 : Sum  Inputs=|+-
  Sum4 : Sum  Inputs=+-
  l : Outport
  d_l : Outport  Port=2
  θl : Outport  Port=3
  wires:
  Product2/1 -> d_l/1
  Sqrt/1 -> l/1, Saturation/1  "l"
  Sum1/1 -> Sqrt/1
  Sum2/1 -> Product1/1, Atan2/2, Square1/1
  Sum/1 -> Product/1, Atan2/1, Square/1
  yl/1 -> Sum2/2
  Atan2/1 -> θl/1
  vly/1 -> Product1/2
  xl/1 -> Sum/1
  Constant/1 -> Sum2/1
  Sum3/1 -> Product/2
  Square1/1 -> Sum1/2
  vt/1 -> Sum3/2
  Sum4/1 -> Product2/2
  vlx/1 -> Sum3/1
  xt/1 -> Sum/2
  Square/1 -> Sum1/1
  Product1/1 -> Sum4/2
  Product/1 -> Sum4/1
  Saturation/1 -> Product2/1

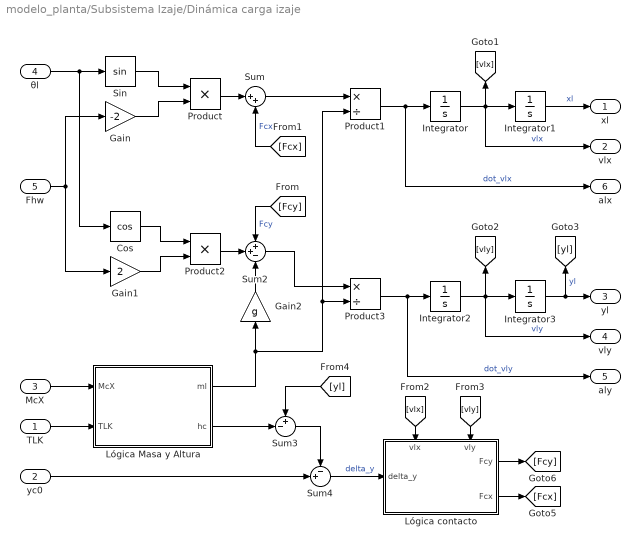
== system modelo_planta/Subsistema Izaje/Dinámica carga izaje ==
  TLK : Inport
  yc0 : Inport  Port=2
  McX : Inport  Port=3
  θl : Inport  Port=4
  Fhw : Inport  Port=5
  Cos : Trigonometry  Operator=cos
  Gain : Gain  Gain=-2
  Gain1 : Gain  Gain=2
  Gain2 : Gain  Gain=g
  Integrator : Integrator  InitialCondition=vlx_0
  Integrator1 : Integrator  InitialCondition=xl_0
  Integrator2 : Integrator  InitialCondition=vly_0
  Integrator3 : Integrator  InitialCondition=yl_0
  Lógica Masa y Altura : Subsystem
  Lógica contacto : Subsystem
      settings: PortSchema="{\"entries\":[{\"content\":{\"sides\":[{\"content\":{\"connectorIds\":[\"In1\"]},\"type\":\"ConnectorPlacement.EquallySpacedRectSide\",\"uuid\":\"20a8b2c4-d5cf-44ce-93ec-929b996a0905\"},{\"content\":{\"connectorIds\":[\"Out1\",\"Out2\"],\"side\":\"RIGHT\"},\"type\":\"ConnectorPlacement.EquallySpacedRectSide\",\"uuid\":\"396e1f2e-cf71-48dc-8d57-a3e2695dfff1\"},{\"content\":{\"connectorIds\":[\"In2\",\"In3\"],\"side\":\"TOP\"},\"type\":\"ConnectorPlacement.EquallySpacedRectSide\",\"uuid\":\"e66c0478-9682-41e1-9b77-d2d789a9c323\"}]},\"type\":\"ConnectorPlacement.EquallySpacedConnector\",\"uuid\":\"193dabd2-f524-433a-b6ef-c1cab585578e\"}],\"packageUris\":[\"http://schema.mathworks.com/mf0/Connector/R2020b\"],\"version\":\"1.0\"}"
  Product : Product
  Product1 : Product  Inputs=*/
  Product2 : Product
  Product3 : Product  Inputs=*/
  Sin : Trigonometry
  Sum : Sum  Inputs=|++
  Sum2 : Sum  Inputs=++-
  Sum3 : Sum  Inputs=+-|
  Sum4 : Sum  Inputs=-+|
  xl : Outport
  vlx : Outport  Port=2
  yl : Outport  Port=3
  vly : Outport  Port=4
  aly : Outport  Port=5
  alx : Outport  Port=6
  wires:
  θl/1 -> Sin/1, Cos/1
  Integrator/1 -> vlx/1, Integrator1/1, [vlx]  "vlx"
  Sum3/1 -> Sum4/1
  Sin/1 -> Product/1
  Gain/1 -> Product/2
  [Fcy] -> Sum2/1  "Fcy"
  Integrator2/1 -> vly/1, Integrator3/1, [vly]  "vly"
  Integrator3/1 -> yl/1, [yl]  "yl"
  Fhw/1 -> Gain1/1, Gain/1
  [Fcx] -> Sum/2  "Fcx"
  Product/1 -> Sum/1
  Product1/1 -> alx/1, Integrator/1  "dot_vlx"
  Gain2/1 -> Sum2/3
  Cos/1 -> Product2/1
  Gain1/1 -> Product2/2
  [yl] -> Sum3/1
  Product2/1 -> Sum2/2
  yc0/1 -> Sum4/2
  Sum2/1 -> Product3/1
  Product3/1 -> aly/1, Integrator2/1  "dot_vly"
  Sum/1 -> Product1/1
  Integrator1/1 -> xl/1  "xl"
  Sum4/1 -> Lógica contacto/1(delta_y)  "delta_y"
  Lógica contacto/1(Fcy) -> [Fcy]
  Lógica contacto/2(Fcx) -> [Fcx]
  Lógica Masa y Altura/1(ml) -> Product1/2, Product3/2, Gain2/1
  McX/1 -> Lógica Masa y Altura/1(McX)
  TLK/1 -> Lógica Masa y Altura/2(TLK)
  Lógica Masa y Altura/2(hc) -> Sum3/2
  [vlx] -> Lógica contacto/2(vlx)
  [vly] -> Lógica contacto/3(vly)

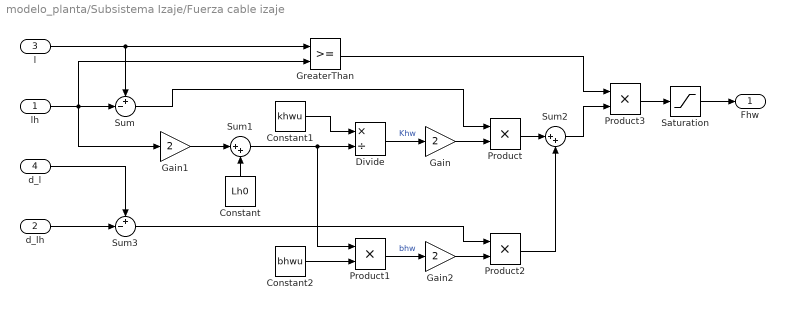
== system modelo_planta/Subsistema Izaje/Fuerza cable izaje ==
  lh : Inport
  d_lh : Inport  Port=2
  l : Inport  Port=3
  d_l : Inport  Port=4
  Constant : Constant  Value=Lh0
  Constant1 : Constant  Value=khwu
  Constant2 : Constant  Value=bhwu
  Divide : Product  Inputs=*/  RndMeth=Zero  SaturateOnIntegerOverflow=on
  Gain : Gain  Gain=2
  Gain1 : Gain  Gain=2
  Gain2 : Gain  Gain=2
  GreaterThan : RelationalOperator  OutDataTypeStr=boolean  RndMeth=Simplest  InputSameDT=off
  Product{,1..3} (4 alike) : Product
  Saturation : Saturate  UpperLimit=inf  LowerLimit=0
  Sum : Sum  Inputs=+-|
  Sum1 : Sum  Inputs=|++
  Sum2 : Sum  Inputs=|++
  Sum3 : Sum  Inputs=+-|
  Fhw : Outport
  wires:
  Constant/1 -> Sum1/2
  Constant2/1 -> Product1/2
  Sum1/1 -> Divide/2, Product1/1
  lh/1 -> Sum/2, GreaterThan/2, Gain1/1
  Product/1 -> Sum2/1
  Gain1/1 -> Sum1/1
  l/1 -> Sum/1, GreaterThan/1
  Product2/1 -> Sum2/2
  Product3/1 -> Saturation/1
  GreaterThan/1 -> Product3/1
  d_lh/1 -> Sum3/2
  Constant1/1 -> Divide/1
  Product1/1 -> Gain2/1  "bhw"
  Sum/1 -> Product/1
  Gain2/1 -> Product2/2
  Divide/1 -> Gain/1  "Khw"
  Sum2/1 -> Product3/2
  Sum3/1 -> Product2/1
  d_l/1 -> Sum3/1
  Gain/1 -> Product/2
  Saturation/1 -> Fhw/1

== system modelo_planta/Subsistema Carro/Accionamiento carro/Freno Motor ==
  BRK_t : Inport
  wtm : Inport  Port=2
  Constant : Constant  Value=0
  Gain3 : Gain  Gain=-Ttb_Max
  Gain4 : Gain  Gain=btb
  Switch : Switch  Criteria=u2 > Threshold  SaturateOnIntegerOverflow=off  InputSameDT=off
  Tanh : Trigonometry  Operator=tanh
  Ttb : Outport
  wires:
  BRK_t/1 -> Switch/2
  Constant/1 -> Switch/1
  wtm/1 -> Gain4/1
  Gain4/1 -> Tanh/1
  Tanh/1 -> Gain3/1
  Gain3/1 -> Switch/3
  Switch/1 -> Ttb/1

== system modelo_planta/Subsistema Izaje/Accionamiento izaje/Freno Emergencia (Drum) ==
  BRK_hE : Inport
  whd : Inport  Port=2
  Constant : Constant  Value=0
  Gain3 : Gain  Gain=-ThEb_Max
  Gain4 : Gain  Gain=bhEb
  Switch : Switch  Criteria=u2 > Threshold  SaturateOnIntegerOverflow=off  InputSameDT=off
  Tanh : Trigonometry  Operator=tanh
  ThEb : Outport
  wires:
  BRK_hE/1 -> Switch/2
  Gain3/1 -> Switch/3
  Constant/1 -> Switch/1
  whd/1 -> Gain4/1
  Gain4/1 -> Tanh/1
  Tanh/1 -> Gain3/1
  Switch/1 -> ThEb/1

== system modelo_planta/Subsistema Izaje/Accionamiento izaje/Freno Motor ==
  BRK_h : Inport
  whm : Inport  Port=2
  Constant : Constant  Value=0
  Gain3 : Gain  Gain=-Thb_Max
  Gain4 : Gain  Gain=bhb
  Switch : Switch  Criteria=u2 > Threshold  SaturateOnIntegerOverflow=off  InputSameDT=off
  Tanh : Trigonometry  Operator=tanh
  Thb : Outport
  wires:
  BRK_h/1 -> Switch/2
  Gain3/1 -> Switch/3
  Constant/1 -> Switch/1
  whm/1 -> Gain4/1
  Gain4/1 -> Tanh/1
  Tanh/1 -> Gain3/1
  Switch/1 -> Thb/1

== system modelo_planta/Subsistema Izaje/Dinámica carga izaje/Lógica Masa y Altura ==
  McX : Inport
  TLK : Inport  Port=2
  Constant : Constant  Value=Ms
  Constant1 : Constant  Value=0
  Constant2 : Constant  Value=Hc
  Rate Limiter : RateLimiter  Commented=through  RisingSlewLimit=Mc_max/0.1  FallingSlewLimit=-Mc_max/0.1  SampleTimeMode=inherited  InitialCondition=Ms
  Sum1 : Sum  Inputs=|++
  Switch : Switch  Criteria=u2 > Threshold  SaturateOnIntegerOverflow=off  InputSameDT=off
  Switch1 : Switch  Criteria=u2 > Threshold  SaturateOnIntegerOverflow=off  InputSameDT=off
  ml : Outport
  hc : Outport  Port=2
  wires:
  Sum1/1 -> Switch/1
  Constant2/1 -> Switch1/1
  TLK/1 -> Switch1/2, Switch/2
  Constant/1 -> Switch/3, Sum1/2
  Constant1/1 -> Switch1/3
  McX/1 -> Sum1/1
  Switch/1 -> Rate Limiter/1
  Rate Limiter/1 -> ml/1
  Switch1/1 -> hc/1

== system modelo_planta/Subsistema Izaje/Dinámica carga izaje/Lógica contacto ==
  delta_y : Inport
  vlx : Inport  Port=2
  vly : Inport  Port=3
  Constant3 : Constant  Value=0
  Constant4 : Constant  Value=0
  Gain3 : Gain  Gain=Kcy
  Gain4 : Gain  Gain=bcy
  Gain5 : Gain  Gain=-bcx
  Saturation : Saturate  UpperLimit=inf  LowerLimit=0
  Sum5 : Sum  Inputs=-+|
  Switch2 : Switch  SaturateOnIntegerOverflow=off  InputSameDT=off
  Switch3 : Switch  SaturateOnIntegerOverflow=off  InputSameDT=off
  Fcy : Outport
  Fcx : Outport  Port=2
  wires:
  Sum5/1 -> Switch2/1
  vlx/1 -> Gain5/1
  Gain4/1 -> Sum5/1
  vly/1 -> Gain4/1
  Constant4/1 -> Switch3/3
  Gain5/1 -> Switch3/1
  Gain3/1 -> Sum5/2
  delta_y/1 -> Switch3/2, Gain3/1, Switch2/2
  Constant3/1 -> Switch2/3
  Switch2/1 -> Saturation/1  "Fcy"
  Switch3/1 -> Fcx/1  "Fcx"
  Saturation/1 -> Fcy/1

== matlab function modelo_planta/Controlador Carro/Control de Balanceo/Factor de Seguridad ==
  data: theta_rad input; g_ang output
function g_ang = ganancia_angular(theta_rad)
    theta_deg = abs(theta_rad * 180 / pi);
    
    L_nominal = 1;  % Ganancia suave para seguir referencia (Zonas < 5°)
    L_agresiva = 2; % Ganancia fuerte para frenar oscilación extrema (Zonas > 15°)
    
    if theta_deg <= 5.0
        % ZONA 1: Viaje suave y parada precisa (+/- 5 grados)
        g_ang = L_nominal;
        
    elseif theta_deg >= 15.0
        % ZONA 3: Emergencia / Aceleración fuerte (+/- 20 grados)
        g_ang = L_agresiva;
        
    else
        % ZONA 2: Transición (Entre 5° y 15°)
        % Interpolación lineal para no dar saltos bruscos en el control
        slope = (L_agresiva - L_nominal) / (15.0 - 5.0);
        g_ang = L_nominal + (theta_deg - 5.0) * slope;
    end
end

== matlab function modelo_planta/Controlador Carro/Control de Balanceo/Compensación de Inercia ==
  data: m_est input; g_masa output; Ms parameter; Mc_max parameter
function g_masa = ganancia_masa(m_est, Ms, Mc_max)
    L_vacio = 1;  % Ganancia actual
    L_lleno = 1.6;  % Gana más agresiva para carga pesada (orig 1.4)
    
    % Factor de carga (0.0 = Vacío, 1.0 = Lleno)
    factor = (m_est - Ms) / Mc_max;
    
    % Saturación por seguridad (0 a 1)
    factor = max(0, min(1, factor));
    
    % Interpolación Lineal
    g_masa = L_vacio + (L_lleno - L_vacio) * factor;
end

== matlab function modelo_planta/MATLAB Function ==
  data: TLK input; M_carga output; Mc_max parameter; Mc_min parameter
function M_carga = Generar_Masa_Aleatoria(TLK, Mc_max, Mc_min)
    persistent masa_actual;
    persistent ultimo_estado_trigger;
    
    % Inicialización
    if isempty(masa_actual)
        masa_actual = Mc_min; % Empezamos con el valor mínimo por defecto
        ultimo_estado_trigger = 0;
    end
    
    % DETECCIÓN DE FLANCO DE SUBIDA (Rising Edge)
    if (TLK == 1 && ultimo_estado_trigger == 0)
        % Generar número aleatorio entre Min y Max
        masa_actual = Mc_min + (Mc_max - Mc_min) * rand();
        masa_actual = floor(masa_actual); 
    end
    
    % Actualizar memoria del trigger
    ultimo_estado_trigger = TLK;
    % Salida: La masa se mantiene constante hasta el próximo trigger
    M_carga = masa_actual;
end

== matlab function modelo_planta/Controlador Carro/Curva S/MATLAB Function ==
  data: error_pos input; vt_cmd output; at_max parameter
function vt_cmd = Frenado_OptimoT(error_pos, at_max)
    % Parámetro de suavizado (región lineal)
    d_tol = 0.1; % 10 cm de tolerancia donde se vuelve lineal
    
    if abs(error_pos) > d_tol
        % ZONA PARABÓLICA (Frenado Óptimo)
        % Lejos del objetivo, usamos la raíz cuadrada
        vh_brakes = sqrt(2 * at_max * abs(error_pos));
        vt_cmd = vh_brakes * sign(error_pos);
    else
        % ZONA LINEAL (Aterrizaje Suave)
        % Cerca del cero, usamos una ganancia fija para evitar pendiente infinita.
        vh_limit_tol = sqrt(2 * at_max * d_tol); % Velocidad en el borde de la zona
        gain_linear = vh_limit_tol / d_tol;      % Pendiente equivalente        
        vt_cmd = gain_linear * error_pos;
    end
end

== matlab function modelo_planta/Controlador Izaje/Curva S/MATLAB Function ==
  data: error_pos input; vh_cmd output; ah_max parameter
function vh_cmd = Frenado_Optimo(error_pos, ah_max)
    % Parámetro de suavizado (región lineal)
    d_tol = 0.1; % 10 cm de tolerancia donde se vuelve lineal

    if abs(error_pos) > d_tol
        % ZONA PARABÓLICA (Frenado Óptimo)
        % Lejos del objetivo, usamos la raíz cuadrada
        vh_brakes = sqrt(2 * ah_max * abs(error_pos));
        vh_cmd = vh_brakes * sign(error_pos);
    else
        % ZONA LINEAL (Aterrizaje Suave)
        % Cerca del cero, usamos una ganancia fija para evitar pendiente infinita.
        vh_limit_tol = sqrt(2 * ah_max * d_tol); % Velocidad en el borde de la zona
        gain_linear = vh_limit_tol / d_tol;      % Pendiente equivalente        
        vh_cmd = gain_linear * error_pos;
    end
end
